simulink model "TestSinglePV"  (R2016b)
settings: Solver=VariableStepAuto  StartTime=0.0  StopTime=2  RelTol=1e-3
libraries: simulink x1
settings Model: Creator=ThinkPad  LastModifiedBy=ThinkPad

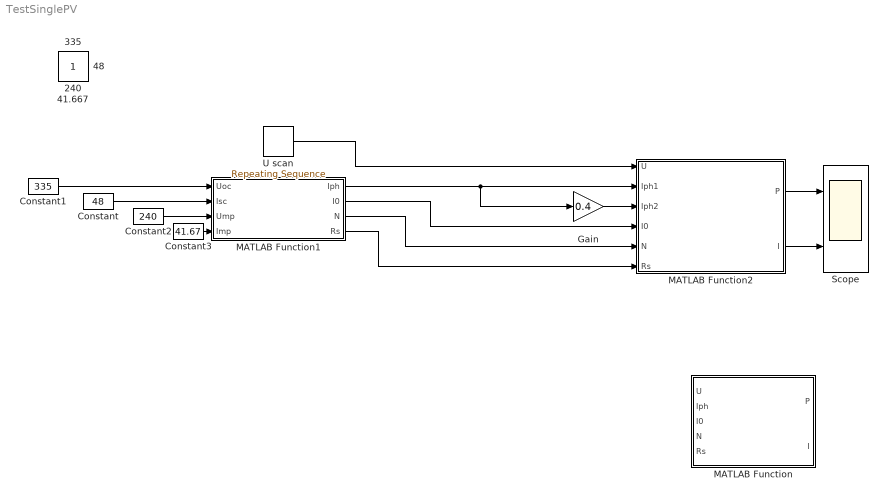
== system TestSinglePV ==
  Constant : Constant  Value=48
  Constant1 : Constant  Value=335
  Constant2 : Constant  Value=240
  Constant3 : Constant  Value=41.67
  Gain : Gain  Gain=0.4
  MATLAB Function : MATLAB Function  TreatAsAtomicUnit=on
  MATLAB Function1 : MATLAB Function  TreatAsAtomicUnit=on
  MATLAB Function2 : MATLAB Function  TreatAsAtomicUnit=on
  Scope : Scope  NumInputPorts=2
  U scan : simulink/Sources/Repeating Sequence  rep_seq_t=[0 1 2]  rep_seq_y=[-50 335 -50]
  240 : Constant  IOType=siggen
  335 : Constant  IOType=siggen
  41.667 : Constant  IOType=siggen
  48 : Constant  IOType=siggen
  wires:
  U scan/1 -> MATLAB Function2/1(U)
  Constant/1 -> MATLAB Function1/2(Isc)
  Constant2/1 -> MATLAB Function1/3(Ump)
  Constant1/1 -> MATLAB Function1/1(Uoc)
  Constant3/1 -> MATLAB Function1/4(Imp)
  MATLAB Function1/1(Iph) -> Gain/1, MATLAB Function2/2(Iph1)
  MATLAB Function1/2(I0) -> MATLAB Function2/4(I0)
  MATLAB Function1/3(N) -> MATLAB Function2/5(N)
  MATLAB Function1/4(Rs) -> MATLAB Function2/6(Rs)
  MATLAB Function2/2(I) -> Scope/2
  MATLAB Function2/1(P) -> Scope/1
  Gain/1 -> MATLAB Function2/3(Iph2)

== matlab function TestSinglePV/MATLAB Function1 ==
  data: Uoc input; Iph output; Isc input; Ump input; Imp input; I0 output; N output; Rs output
function [Iph, I0, N, Rs] = calcPvParameters(Uoc, Isc, Ump, Imp)
Iph = Isc;
N = (Imp-Isc)*(2*Ump-Uoc)/(-Imp+(Imp-Isc)*log(1-Imp/Isc));
Rs=Ump/Imp+(2*Ump-Uoc)/(-Imp+(Imp-Isc)*log(1-Imp/Isc));
I0=Iph*exp(-Uoc/N);
end

== matlab function TestSinglePV/MATLAB Function ==
  data: P output; U input; Iph input; I output; I0 input; N input; Rs input
function [P,I] = PvFunctionI(U,Iph,I0,N,Rs)
eps = 1e-5;
I = Iph;
f = U+I*Rs-N*log((I0+Iph-I)/I0);
while(abs(f) > eps)    
    I = I - f/(Rs + N/(I0 - I + Iph));
    f = U+I*Rs-N*log((I0+Iph-I)/I0);
end
I = I + I0*(exp(-10/N*U)-1);
P = U * I;
end

== matlab function TestSinglePV/MATLAB Function2 ==
  data: U input; Iph1 input; P output; Iph2 input; I0 input; N input; Rs input; I output
function [P,I] = Pv2Series(U,Iph1,Iph2,I0,N,Rs)
coder.extrinsic('fsolve');
dI=@(u1) PvFunctionI(u1,Iph1,I0,N,Rs)-PvFunctionI(U-u1,Iph2,I0,N,Rs);

U1=fsolve(dI,U,optimset('Display','off'));
I=PvFunctionI(U1,Iph1,I0,N,Rs);
P=U*I;
end
